simulink model "LQG_AWBT_backup"  (R2015a)
settings: Solver=ode5  StartTime=0.0  StopTime=0.5  FixedStep=1e-4  RelTol=1e-3
values from neighbouring files (symbols this model uses):
  Lambda = X/M    [main_matlab.m]
  nk = sqrt(numel(Ak))    [main_matlab.m]
  nu = numel(Bpu)/np    [main_matlab.m]
undefined symbols (not defined in the file or in its folder): Af, Bf, Cf, Hf
libraries: cstblocks x2, simulink x1
settings Model: Creator=p4wp4w  LastModifiedBy=Ablah

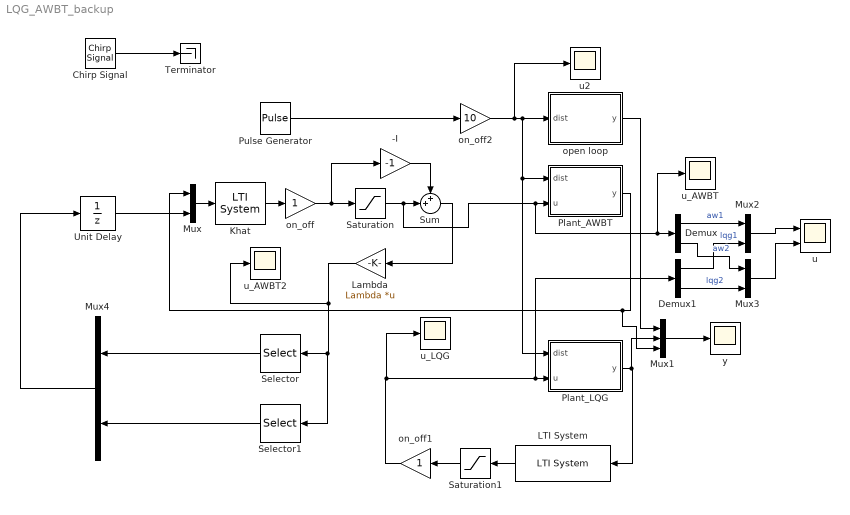
== system LQG_AWBT_backup ==
  -I : Gain  Gain=-1
  Chirp Signal : simulink/Sources/Chirp Signal  f1=0.1  T=10  f2=800
  Demux : Demux  Outputs=2
  Demux1 : Demux  Outputs=2
  Khat : cstblocks/LTI System  sys=Khat  IC=[]
  LTI System : cstblocks/LTI System  sys=rlqg  IC=[]
  Lambda : Gain  Gain=Lambda  Multiplication=Matrix(K*u)
  Mux{,2..4} (4 alike) : Mux  Inputs=2
  Mux1 : Mux  Inputs=3
  Plant_AWBT : Subsystem
  Plant_LQG : Subsystem
  Pulse Generator : DiscretePulseGenerator  PulseType=Time based  Period=0.5  PulseWidth=10
  Saturation : Saturate  UpperLimit=2  LowerLimit=-2
  Saturation1 : Saturate  UpperLimit=2  LowerLimit=-2
  Selector : Selector  InputPortWidth=nk+nu  Indices=[1:nk]
  Selector1 : Selector  InputPortWidth=nk+nu  Indices=[nk+1:nk+nu]
  Sum : Sum  Inputs=++|
  Terminator : Terminator
  Unit Delay : UnitDelay  SampleTime=-1
  on_off : Gain
  on_off1 : Gain
  on_off2 : Gain  Gain=10
  open loop : Subsystem
  u : Scope  NumInputPorts=2
      settings: ShowLegends=on  YMin=-0.8~-5  YMax=0.7~5  SaveName=ScopeData3
  u2 : Scope
      settings: ShowLegends=on  YMin=-0.8  YMax=0.7  SaveName=ScopeData6
  u_AWBT : Scope
      settings: YMin=-1  YMax=1
  u_AWBT2 : Scope
      settings: YMin=-150  YMax=150  SaveName=ScopeData4
  u_LQG : Scope
      settings: SaveName=ScopeData2
  y : Scope
      settings: ShowLegends=on  YMin=-15  YMax=15
  wires:
  Khat/1 -> on_off/1
  Saturation/1 -> Sum/2, u_AWBT/1, Demux/1, Plant_AWBT/2(u)
  on_off/1 -> -I/1, Saturation/1
  LTI System/1 -> Saturation1/1
  Saturation1/1 -> on_off1/1
  Mux1/1 -> y/1
  open loop/1(y) -> Mux1/1
  on_off1/1 -> u_LQG/1, Demux1/1, Plant_LQG/2(u)
  Lambda/1 -> Selector1/1, Selector/1, u_AWBT2/1
  Mux/1 -> Khat/1
  Mux4/1 -> Unit Delay/1
  -I/1 -> Sum/1
  Sum/1 -> Lambda/1
  on_off2/1 -> u2/1, open loop/1(dist), Plant_LQG/1(dist), Plant_AWBT/1(dist)
  Plant_LQG/1(y) -> Mux1/2, LTI System/1
  Plant_AWBT/1(y) -> Mux1/3, Mux/1
  Selector/1 -> Mux4/1
  Demux/1 -> Mux2/1  "aw1"
  Demux1/1 -> Mux2/2  "lqg1"
  Demux/2 -> Mux3/1  "aw2"
  Demux1/2 -> Mux3/2  "lqg2"
  Chirp Signal/1 -> Terminator/1
  Pulse Generator/1 -> on_off2/1
  Mux2/1 -> u/1
  Mux3/1 -> u/2
  Selector1/1 -> Mux4/2
  Unit Delay/1 -> Mux/2

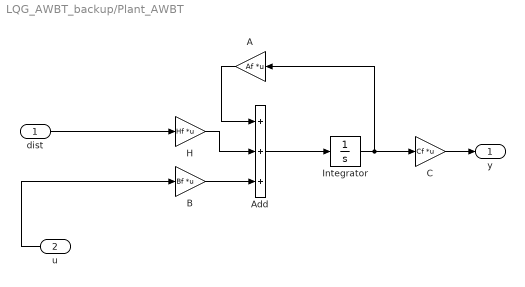
== system LQG_AWBT_backup/Plant_AWBT ==
  dist : Inport
  u : Inport  Port=2
  A : Gain  Gain=Af  Multiplication=Matrix(K*u)
  Add : Sum  Inputs=+++
  B : Gain  Gain=Bf  Multiplication=Matrix(K*u)
  C : Gain  Gain=Cf  Multiplication=Matrix(K*u)
  H : Gain  Gain=Hf  Multiplication=Matrix(K*u)
  Integrator : Integrator
  y : Outport
  wires:
  Add/1 -> Integrator/1
  H/1 -> Add/2
  A/1 -> Add/1
  dist/1 -> H/1
  C/1 -> y/1
  B/1 -> Add/3
  Integrator/1 -> C/1, A/1
  u/1 -> B/1

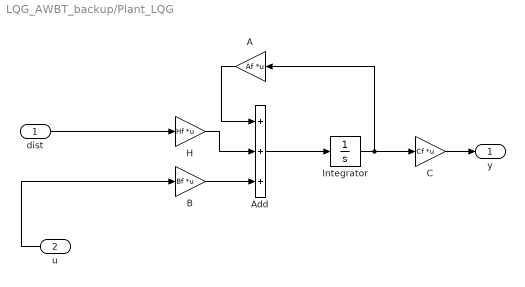
== system LQG_AWBT_backup/Plant_LQG ==
  dist : Inport
  u : Inport  Port=2
  A : Gain  Gain=Af  Multiplication=Matrix(K*u)
  Add : Sum  Inputs=+++
  B : Gain  Gain=Bf  Multiplication=Matrix(K*u)
  C : Gain  Gain=Cf  Multiplication=Matrix(K*u)
  H : Gain  Gain=Hf  Multiplication=Matrix(K*u)
  Integrator : Integrator
  y : Outport
  wires:
  u/1 -> B/1
  Integrator/1 -> A/1, C/1
  B/1 -> Add/3
  C/1 -> y/1
  dist/1 -> H/1
  A/1 -> Add/1
  H/1 -> Add/2
  Add/1 -> Integrator/1

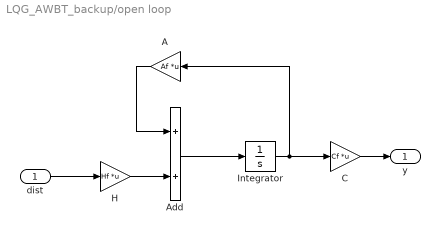
== system LQG_AWBT_backup/open loop ==
  dist : Inport
  A : Gain  Gain=Af  Multiplication=Matrix(K*u)
  Add : Sum
  C : Gain  Gain=Cf  Multiplication=Matrix(K*u)
  H : Gain  Gain=Hf  Multiplication=Matrix(K*u)
  Integrator : Integrator
  y : Outport
  wires:
  Integrator/1 -> A/1, C/1
  C/1 -> y/1
  dist/1 -> H/1
  A/1 -> Add/1
  H/1 -> Add/2
  Add/1 -> Integrator/1
